simulink model "lut_example_1d"  (R2020b)
settings: Solver=VariableStepAuto  StartTime=0.0  StopTime=10.0  RelTol=1e-3
settings Model: Creator=abdullah  LastModifiedBy=abdullah

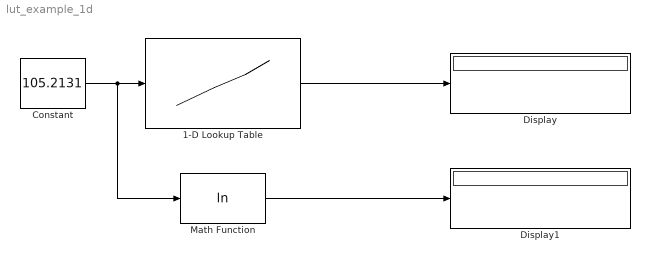
== system lut_example_1d ==
  1-D Lookup Table : Lookup_n-D  NumberOfTableDimensions=1  BreakpointsForDimension1=[0.5:0.5:15]  Table=log([0.5:0.5:15])  InternalRulePriority=Speed  RndMeth=Simplest  InputSameDT=on
  Constant : Constant  Value=105.2131
  Display : Display
  Display1 : Display
  Math Function : Math  Operator=log  SaturateOnIntegerOverflow=on
  wires:
  Constant/1 -> Math Function/1, 1-D Lookup Table/1
  1-D Lookup Table/1 -> Display/1
  Math Function/1 -> Display1/1
